simulink model "ADCS_MIL"  (R2024a)
settings: Solver=FixedStepAuto  StartTime=0.0  StopTime=6000  RelTol=1e-3
undefined symbols (not defined in the file or in its folder): agh, attitude, Cd, dgh, Eearth, epoch, Esun, Jsc, juliandate, k_Bdot, Kd1, Kd2, Kd3, km, Kp1, Kp2, Kp3, m, m_disturb, MTQ_Swithces, NoiseStd, s, satellite, signQuat, simulator, Surf_areas, Surf_dist, Surf_normals, Surf_reflectivity, WMM2020
libraries: sharedtransform x18, aerolibconvert2 x12, SepehrMILLib x11, simulink_extras x8, aerolibsatdyn x5, aerolibutil x5, sharedutil x3, vrlib x3, aerolibtransform2 x3, aerolibgravity2 x3, matrix_library x2
(part 1 of 3)
settings Model: Creator=dani  LastModifiedBy=dani

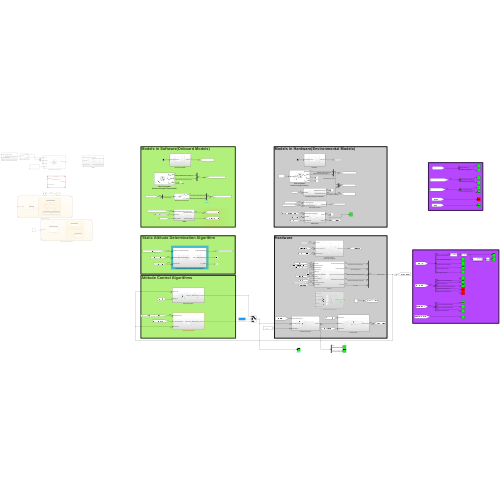
[thumbnail: Simulink's stored preview of the top-level diagram]
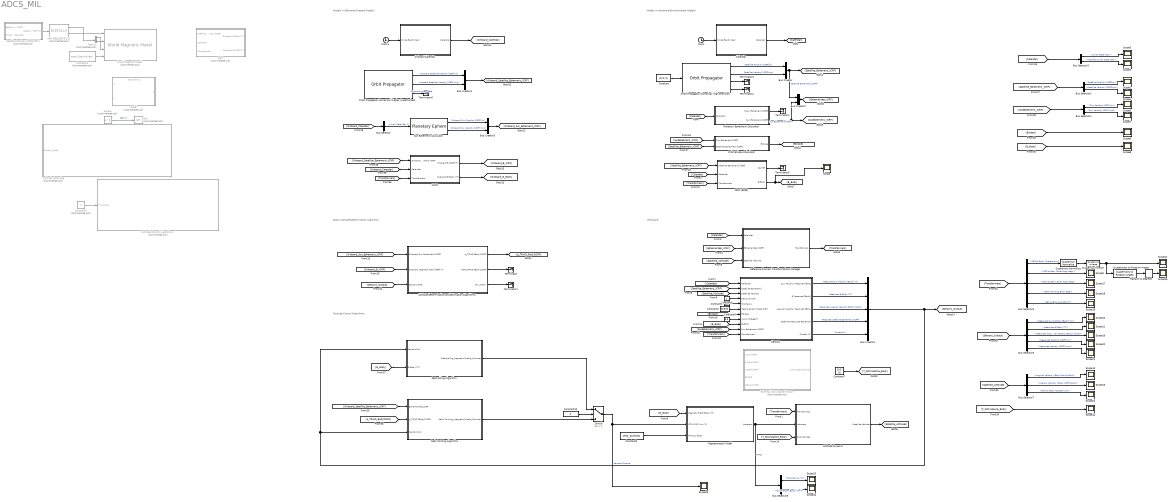
== system ADCS_MIL ==
  note: Hardware
  note: Models in Software(Onboard Models)
  note: Static Attitude Determination Algorithm
  note: Attitude Control Algorithms
  note: Models in Hardware(Environmental Models)
  Attitude Control Algorithms : Stateflow chart  Commented=on  TreatAsAtomicUnit=on
  Attitude Controlgg : Stateflow chart  Commented=on  TreatAsAtomicUnit=on
  Attitude Determination and Estimation Algorithms : Subsystem
  Attitude Dynamic : Subsystem
  Bus Creator{,2..4} (4 alike) : BusCreator  Inputs=2
  Bus Creator1 : BusCreator  Inputs=5
  Bus Selector : BusSelector  OutputSignals=Julian Date (day)
  Bus Selector2 : BusSelector  OutputSignals=Satellite Position [ICRF](m),Satellite Velocity [ICRF](m/s)
  Bus Selector3 : BusSelector  OutputSignals=Julian Date (day),Modified Julian Date (day)
  Bus Selector4 : BusSelector  OutputSignals=Sun Position [ICRF] (m),Sun Velocity [ICRF] (m/s)
  Bus Selector5 : BusSelector  OutputSignals=Measured Sun Position [Body] (m),Measured B [Body] (T),Measured Angular Velocity [Body] (rad/s),Measured Satellite Ephemeris [ICRF].Measured Position [ICRF] (m),Measured Satellite Ephemeris [ICRF].Measured Velocity [ICRF] (m/s)
  Bus Selector6 : BusSelector  OutputSignals=Quaternions.ICRF to Body Quaternions,Euler Angles (deg).ICRF to Body Euler Angs (deg),Euler Angles (deg).Orbit to Body Euler Angs (deg),Pinting Error (Deg).Nadir Pointing Error (deg),Orbital Elements.Semi-Major Axis [a] (m)
  Bus Selector7 : BusSelector  OutputSignals=Angular Velocity {Body-Orbit}(rad/s),Angular Velocity {Body-ICRF}(rad/s),Orbit to Body Quaternions
  Bus Selector8 : BusSelector  OutputSignals=Dipoles (Am^2),CoilsTorque [Body] (Nm)
  "Calendar " : Subsystem
  Clock : Clock
  Clock1 : Clock
  Constant : Constant  Value=[0; 0; 0]
  Constant1 : Constant  Value=20
  Constant10 : Constant  Value=0
  Constant2 : Constant  Value=eye(3)
  Constant3 : Constant  Commented=on  Value=epoch.DecimalYear
  Constant4 : Constant  Commented=on  Value=2
  Constant5 : Constant
  Constant6 : Constant  Value=3.3
  Constant7 : Constant  Value=[0 0 0]
  Constant9 : Constant  Value=MTQ_Swithces
  Demux : Demux  Commented=on  Outputs=2
  Detumbling Algorithm : Subsystem
  External Disturbance Torque : Subsystem  Commented=on
  IGRF : Subsystem  Commented=on
  IGRF [ECEF] : Subsystem
  ITRF Position to LLA : ECEF2LLA  Commented=on
  Magnetorquers Model : Subsystem
  Model : ModelReference  Commented=on  ModelNameDialog=Detumbling.slx  SimulationMode=Normal  ModelReferenceVersion=1.5
      settings: PortSchema="{\"entries\":[{\"content\":{\"sides\":[{\"content\":{\"connectorIds\":[\"In2\",\"In1\"]},\"type\":\"ConnectorPlacement.EquallySpacedRectSide\",\"uuid\":\"6955eca1-02f6-4ce4-b58e-cf6f86409957\"},{\"content\":{\"connectorIds\":[\"Out1\"],\"side\":\"RIGHT\"},\"type\":\"ConnectorPlacement.EquallySpacedRectSide\",\"uuid\":\"f24cf38f-2c71-460d-85e4-067bf27b1853\"},{\"content\":{\"side\":\"TOP\"},\"type\":\"ConnectorPlacement.EquallySpacedRectSide\",\"uuid\":\"bfc76406-ab18-49d9-8c0b-a4b5f97489f3\"}]},\"type\":\"ConnectorPlacement.EquallySpacedConnector\",\"uuid\":\"b367625e-d4b0-440c-86d9-252cf79ffd42\"}],\"packageUris\":[\"http://schema.mathworks.com/mf0/Connector/R2020b\"],\"version\":\"1.0\"}"
  Nadir Pointing Algorithm : Subsystem
  Onboard Calendar : Subsystem
  Orbit Eclipse Calculator : Subsystem
  Orbit Propagator Numerical (Kepler-Unperturbed) : OrbitPropagator  accelIn=on  startDate=juliandate(epoch.Year, epoch.Month, epoch.Day, epoch.Hour, epoch.Minute, epoch.Second)  orbitType=Circular inclined  semiMajorAxis=Semi_major_axis  inclination=Inclination  raan=RAAN  argLat=Argument_of_latitude  inertialPosition=[3649700.0 3308200.0 -4676600.0]  inertialVelocity=[-2750.8 6666.4 2573.4]  fixedPosition=[-4142689.0 -2676864.7 -4669861.6]  fixedVelocity=[1452.7 -6720.7 2568.1]  customR=3396200  customMu=4.305e13  customJ2=1.0826269e-03  customOmega=4.06125949e-3  outputTransform=on
  Orbit Propagator Numerical (high precision) : OrbitPropagator  propagator=Numerical (high precision)  accelIn=on  startDate=juliandate(epoch.Year, epoch.Month, epoch.Day, epoch.Hour, epoch.Minute, epoch.Second)  orbitType=Circular inclined  semiMajorAxis=Semi_major_axis  inclination=Inclination  raan=RAAN  argLat=Argument_of_latitude  inertialPosition=[3649700.0 3308200.0 -4676600.0]  inertialVelocity=[-2750.8 6666.4 2573.4]  fixedPosition=[-4142689.0 -2676864.7 -4669861.6]  fixedVelocity=[1452.7 -6720.7 2568.1]  customR=3396200  customMu=4.305e13  customJ2=1.0826269e-03  customOmega=4.06125949e-3  outputTransform=on
  Planetary Ephemeris Calculator : Subsystem
  Quaternion Inverse : aerolibutil/Quaternion Inverse
  Quaternion Normalize : sharedutil/Quaternion Normalize  aMode=aMode
  Quaternions to Rotation Angles : sharedtransform/Quaternions to Rotation Angles  rotationOrder=XYZ  aMode=aMode
  Radians to Degrees : simulink_extras/Transformations/Radians to Degrees
  Reference Frames Transformations Manager : Subsystem
  Satellite Position [ICRF2ITRF] : Subsystem  Commented=on
  Scope{,1..26} (27 alike) : Scope
  Sensors : Subsystem
  Sqrt : Sqrt  Commented=on
  Square : Math  Commented=on  Operator=square
  Sun Ephemeris Calculator : PlanetaryEphem  target=Sun
  Switch : Switch  Criteria=u2 > Threshold  Threshold=1  SaturateOnIntegerOverflow=off  InputSameDT=off
  Terminator{,1..6} (7 alike) : Terminator
  WMM : Subsystem
  World Magnetic Model : aerolibgravity2/World Magnetic Model  Commented=on  model=WMM2020 (2020-2025)  customFile='WMM2020.COF'  units=Metric (MKS)  time_in=on  month=January  day=1  year=2020  action=Error  h_out=off  dec_out=off  inc_out=off  ti_out=off
  wires:
  [Calendar] -> Sensors/1(Calendar)
  [Transformers] -> IGRF [ECEF]/3(Transformers)
  [Calendar] -> IGRF [ECEF]/2(Calendar)
  [Satellite_Attitude] -> Reference Frames Transformations Manager/3(Satellite Attitude)
  Sensors/2(B Measured [Body]) -> Bus Creator1/2  "Measured B [Body] (T)"
  Constant5/1 -> Sensors/4(Sensor Switch)
  [Ephemerides_ICRF] -> Reference Frames Transformations Manager/2(Ephemerides [ICRF])
  Attitude Dynamic/1(Satellite Attitude) -> [Satellite_Attitude]
  Constant9/1 -> Magnetorquers Model/3(MTQ Switches)
  [B_Body] -> Magnetorquers Model/1(Magnetic Field [Body] (T))
  Sensors/4(Satellite Measured Ephemeris) -> Bus Creator1/4  "Measured Satellite Ephemeris [ICRF]"
  Magnetorquers Model/1(Acutators) -> Bus Selector8/1, Attitude Dynamic/2(Actuators)  "MTQs"
  Sensors/3(Angular Velocity Measured [Body]) -> Bus Creator1/3  "Measured Angular Velocity [Body] (rad/s)"
  Sensors/1(Sun Position Measured [Body]) -> Bus Creator1/1  "Measured Sun Position [Body] (m)"
  "Calendar "/1(Calendar) -> [Calendar]
  Clock/1 -> "Calendar "/1(Since Epoch (sec))
  Reference Frames Transformations Manager/1(Transformers) -> [Transformers]
  Orbit Propagator Numerical (high precision)/2 -> Bus Creator/2  "Satellite Velocity [ICRF](m/s)"
  [Calendar] -> Planetary Ephemeris Calculator/1(Calendar)
  Orbit Propagator Numerical (high precision)/1 -> Bus Creator/1  "Satellite Position [ICRF](m)"
  Planetary Ephemeris Calculator/2(Sun Ephemeris [ICRF]) -> Bus Creator2/2, [SunEphemeris_ICRF]  "Sun Ephemeris [ICRF]"
  [Calendar] -> Reference Frames Transformations Manager/1(Calendar)
  Planetary Ephemeris Calculator/1(Moon Ephemeris [ICRF]) -> Terminator4/1
  [Transformers] -> Attitude Dynamic/1(Transformers)
  Constant7/1 -> [T_Distrubance_Body]
  Orbit Propagator Numerical (high precision)/4 -> Terminator2/1
  Constant1/1 -> Sensors/5(MM_Temp)
  [Satellite_Attitude] -> Sensors/3(Satellite Attitude)
  Constant2/1 -> Sensors/6(Measurement Model DCM)
  Constant/1 -> Orbit Propagator Numerical (high precision)/1
  [Satellite_Ephemeris_ICRF] -> Sensors/2(Satellite Ephemeris)
  Sensors/5(Current (A)) -> Bus Creator1/5  "Current (A)"
  [Eclipse] -> Sensors/7(Eclipse)
  [T_Distrubance_Body] -> Attitude Dynamic/3(Disturbances)
  Bus Creator1/1 -> [Sensors_Output], Detumbling Algorithm/1(Sensors Out), Nadir Pointing Algorithm/3(Sensors Out)  "Sensors Outputs"
  Orbit Propagator Numerical (high precision)/3 -> Terminator3/1
  Orbit Propagator Numerical (Kepler-Unperturbed)/1 -> Bus Creator4/1  "Onboard Satellite Position [ICRF] (m)"
  Attitude Determination and Estimation Algorithms/3(Cov_Matrix) -> Terminator1/1
  Attitude Determination and Estimation Algorithms/2(DCM_TRIAD [Body2ICRF]) -> Terminator/1
  Attitude Determination and Estimation Algorithms/1(q_TRIAD [Body2ICRF]) -> [q_TRIAD_Body2ICRF]
  IGRF [ECEF]/2(B_Body) -> Scope/1, [B_Body]
  IGRF [ECEF]/1(B_ITRF) -> Terminator5/1
  [B_Body] -> Sensors/9(B_Body)
  Constant4/1 -> Attitude Control Algorithms/1(Sys_Mode)
  [SunEphemeris_ICRF] -> Orbit Eclipse Calculator/1(Sun Ephemeris [ICRF])
  [Satellite_Ephemeris_ICRF] -> Orbit Eclipse Calculator/2(Satellite Ephemeris [ICRF])
  Orbit Eclipse Calculator/1(Eclipse) -> [Eclipse]
  Bus Creator/1 -> Bus Creator2/1, [Satellite_Ephemeris_ICRF]  "Satellite Ephemeris [ICRF]"
  [Satellite_Ephemeris_ICRF] -> IGRF [ECEF]/1(Satellite Ephemeris [ICRF])
  Bus Creator2/1 -> [Ephemerides_ICRF]
  Constant6/1 -> Sensors/8(Input Voltage(V))
  Sun Ephemeris Calculator/1 -> Bus Creator3/1  "Onboard Sun Position [ICRF] (m)"
  Sun Ephemeris Calculator/2 -> Bus Creator3/2  "Onboard Sun Velocity [ICRF] (m/s)"
  Bus Creator3/1 -> [Onboard_Sun_Ephemeris_ICRF]
  Orbit Propagator Numerical (Kepler-Unperturbed)/2 -> Bus Creator4/2  "Onboard Satellite Velocity [ICRF] (m/s)"
  Bus Creator4/1 -> [Onboard_Satellite_Ephemeris_ICRF]
  [Onboard_Calendar] -> Bus Selector/1
  Bus Selector/1 -> Sun Ephemeris Calculator/1  "<Julian Date (day)>"
  Clock1/1 -> Onboard Calendar/1(Since Epoch (sec))
  Onboard Calendar/1(Calendar) -> [Onboard_Calendar]
  Orbit Propagator Numerical (Kepler-Unperturbed)/3 -> Terminator6/1  "Onboard Julian Date"
  [SunEphemeris_ICRF] -> Sensors/10(Sun Ephemeris [ICRF])
  [Transformers] -> Sensors/11(Transformers)
  [Onboard_Sun_Ephemeris_ICRF] -> Attitude Determination and Estimation Algorithms/1(Onboard Sun Ephemeris [ICRF])
  [Calendar] -> Bus Selector3/1
  [Satellite_Ephemeris_ICRF] -> Bus Selector2/1
  [SunEphemeris_ICRF] -> Bus Selector4/1
  [Eclipse] -> Scope6/1
  Bus Selector3/1 -> Scope3/1  "<Julian Date (day)>"
  Bus Selector3/2 -> Scope1/1  "<Modified Julian Date (day)>"
  Bus Selector2/1 -> Scope2/1  "<Satellite Position [ICRF](m)>"
  Bus Selector2/2 -> Scope4/1  "<Satellite Velocity [ICRF](m/s)>"
  Bus Selector4/2 -> Scope7/1  "<Sun Velocity [ICRF] (m/s)>"
  Bus Selector4/1 -> Scope5/1  "<Sun Position [ICRF] (m)>"
  [B_Body] -> Scope8/1
  Bus Selector6/1 -> Quaternion Normalize/1  "<ICRF to Body Quaternions>"
  Bus Selector6/2 -> Scope9/1  "<ICRF to Body Euler Angs (deg)>"
  [Sensors_Output] -> Bus Selector5/1
  Bus Selector5/2 -> Scope12/1  "<Measured B [Body] (T)>"
  [Satellite_Attitude] -> Bus Selector7/1
  [T_Distrubance_Body] -> Scope14/1
  Bus Selector5/1 -> Scope10/1  "<Measured Sun Position [Body] (m)>"
  [Transformers] -> Bus Selector6/1
  Bus Selector7/1 -> Scope13/1  "<Angular Velocity {Body-Orbit}(rad/s)>"
  Bus Selector7/2 -> Scope15/1  "<Angular Velocity {Body-ICRF}(rad/s)>"
  Bus Selector6/3 -> Scope17/1  "<Orbit to Body Euler Angs (deg)>"
  Bus Selector6/4 -> Scope18/1  "<Nadir Pointing Error (deg)>"
  Bus Selector6/5 -> Scope19/1  "<Semi-Major Axis [a] (m)>"
  Bus Selector5/3 -> Scope16/1  "<Measured Angular Velocity [Body] (rad/s)>"
  Bus Selector5/5 -> Scope21/1  "<Measured Velocity [ICRF] (m/s)>"
  Bus Selector5/4 -> Scope20/1  "<Measured Position [ICRF] (m)>"
  Bus Selector7/3 -> Scope22/1  "<Orbit to Body Quaternions>"
  Square/1 -> Sqrt/1  "||B||^2"
  Bus Selector8/1 -> Scope23/1  "<Dipoles (Am^2)>"
  Bus Selector8/2 -> Scope24/1  "<CoilsTorque [Body] (Nm)>"
  Constant10/1 -> Switch/2
  Switch/1 -> Scope25/1, Magnetorquers Model/2(MTQ CMD (A.m^2))
  Detumbling Algorithm/1(Detumbling_Magnetic Dipole_Command) -> Switch/1
  [Onboard_Satellite_Ephemeris_ICRF] -> Nadir Pointing Algorithm/1(Ephemerides_ICRF)
  [B_Body] -> Detumbling Algorithm/2(B [Body] (T))
  [q_TRIAD_Body2ICRF] -> Nadir Pointing Algorithm/2(q_TRIAD [Body2ICRF])
  Quaternion Normalize/1 -> Quaternion Inverse/1
  Quaternion Inverse/1 -> Quaternions to Rotation Angles/1, Scope11/1
  Quaternions to Rotation Angles/1 -> Radians to Degrees/1
  Radians to Degrees/1 -> Scope26/1
  [Transformers] -> WMM/3(Transformers)
  [Onboard_Calendar] -> WMM/2(Calendar)
  [Onboard_Satellite_Ephemeris_ICRF] -> WMM/1(Onboard Satellite Ephemeris [ICRF])
  ITRF Position to LLA/1 -> Demux/1
  Satellite Position [ICRF2ITRF]/1(Satellite Position [ITRF] (m)) -> ITRF Position to LLA/1
  Demux/2 -> World Magnetic Model/3
  Demux/1 -> World Magnetic Model/2
  ITRF Position to LLA/2 -> World Magnetic Model/1
  Constant3/1 -> World Magnetic Model/4
  WMM/1(Onboard B [ICRF] (T)) -> [Onboard_B_ICRF]
  [Sensors_Output] -> Attitude Determination and Estimation Algorithms/3(Sensors Data)
  [Onboard_B_ICRF] -> Attitude Determination and Estimation Algorithms/2(Onboard Magnetic Field [ICRF] (T))
  WMM/2(Onboard B [Body] (T)) -> [Onboard_B_Body]
  Nadir Pointing Algorithm/1(Nadir Pointing_Magnetic Dipole_Command) -> Switch/3

== system ADCS_MIL/Attitude Control Algorithms/Off ==
  Sys_Mode : Inport
  Action Port : ActionPort
      settings: CopyFcn=Stateflow.SLINSF.SimulinkMan.removeBlockPreDeleteFcn  PreDeleteFcn=Stateflow.SLINSF.SimulinkMan.unsafePredeleteFcn

== system ADCS_MIL/Attitude Control Algorithms/On.Detumbling ==
  Sys_Mode : Inport
  Action Port : ActionPort
      settings: CopyFcn=Stateflow.SLINSF.SimulinkMan.removeBlockPreDeleteFcn  PreDeleteFcn=Stateflow.SLINSF.SimulinkMan.unsafePredeleteFcn
  Model : ModelReference  ModelNameDialog=Detumbling.slx  SimulationMode=Normal  ModelReferenceVersion=1.1
  Terminator : Terminator
  wires:
  Sys_Mode/1 -> Terminator/1

== system ADCS_MIL/Attitude Control Algorithms/On.Nadir_Pointing ==
  Sys_Mode : Inport
  q_TRIAD : Inport  Port=2
  Action Port : ActionPort
      settings: CopyFcn=Stateflow.SLINSF.SimulinkMan.removeBlockPreDeleteFcn  PreDeleteFcn=Stateflow.SLINSF.SimulinkMan.unsafePredeleteFcn

== system ADCS_MIL/Attitude Controlgg/Off ==
  SensorsOut : Inport  OutDataTypeStr=Bus: StatesOutBus
  " " : ActionPort
      settings: CopyFcn=Stateflow.SLINSF.SimulinkMan.removeBlockPreDeleteFcn  PreDeleteFcn=Stateflow.SLINSF.SimulinkMan.unsafePredeleteFcn
  Terminator : Terminator
  TorqueCmds : Constant  Value=[0 0 0]
  Unit quat : Constant  Value=[1 0 0 0]
  PointingCmd : Outport  VectorParamsAs1DForOutWhenUnconnected=off
  cmd_q_b2tgt : Outport  Port=2  VectorParamsAs1DForOutWhenUnconnected=off
  wires:
  SensorsOut/1 -> Terminator/1
  TorqueCmds/1 -> PointingCmd/1  "torque_cmds"
  Unit quat/1 -> cmd_q_b2tgt/1  "torque_cmds"

== system ADCS_MIL/Attitude Controlgg/On.Detumbling ==
  SensorsOut : Inport  OutDataTypeStr=Bus: StatesOutBus
  Environment : Inport  Port=2  OutDataTypeStr=Bus: EnvBus
  " " : ActionPort
      settings: CopyFcn=Stateflow.SLINSF.SimulinkMan.removeBlockPreDeleteFcn  PreDeleteFcn=Stateflow.SLINSF.SimulinkMan.unsafePredeleteFcn
  Attitude Profile (Sun Tracking) : aerolibsatdyn/Attitude Profile (Nadir Pointing)  outputError=on  outputFinalAttitude=off  portFrame=ICRF  pointingMode=Custom  celestialTarget=Sun  tunablePointing=off  primaryAlignmentSrc=Dialog  primaryAlignment=[0 0 -1]  secondaryAlignmentSrc=Dialog  secondaryAlignment=[1 0 0]  constraintFrame=ICRF  primaryConstraintSrc=Port  primaryConstraint=[1 0 0]  secondaryConstraintSrc=Dialog  secondaryConstraint=[0 0 1]
  Bus Selector : BusSelector  OutputSignals=x_sun_eci
  Bus Selector1 : BusSelector  OutputSignals=X_eci,q_eci2b
  Model : ModelReference  ModelNameDialog=Detumbling.slx  SimulationMode=Normal  ModelReferenceVersion=1.1
  Quaternion Conjugate : aerolibutil/Quaternion Conjugate
  Quaternions to Rotation Angles1 : sharedtransform/Quaternions to Rotation Angles  rotationOrder=XYZ  aMode=aMode
  PointingCmd : Outport  VectorParamsAs1DForOutWhenUnconnected=off
  cmd_q_b2tgt : Outport  Port=2  VectorParamsAs1DForOutWhenUnconnected=off
  wires:
  Attitude Profile (Sun Tracking)/1 -> Quaternions to Rotation Angles1/1, cmd_q_b2tgt/1
  SensorsOut/1 -> Bus Selector1/1
  Environment/1 -> Bus Selector/1
  Quaternions to Rotation Angles1/1 -> PointingCmd/1
  Bus Selector/1 -> Attitude Profile (Sun Tracking)/3  "<x_sun_eci>"
  Quaternion Conjugate/1 -> Attitude Profile (Sun Tracking)/2
  Bus Selector1/2 -> Quaternion Conjugate/1  "<q_eci2b>"
  Bus Selector1/1 -> Attitude Profile (Sun Tracking)/1  "<X_eci>"

== system ADCS_MIL/Attitude Controlgg/On.Nadir_Pointing ==
  SensorsOut : Inport  OutDataTypeStr=Bus: StatesOutBus
  " " : ActionPort
      settings: CopyFcn=Stateflow.SLINSF.SimulinkMan.removeBlockPreDeleteFcn  PreDeleteFcn=Stateflow.SLINSF.SimulinkMan.unsafePredeleteFcn
  Attitude Profile (Nadir Pointing) : aerolibsatdyn/Attitude Profile (Nadir Pointing)  outputError=on  outputFinalAttitude=off  portFrame=ICRF  pointingMode=Point at nadir  celestialTarget=Sun  tunablePointing=off  primaryAlignmentSrc=Dialog  primaryAlignment=[0 0 1]  secondaryAlignmentSrc=Dialog  secondaryAlignment=[1 0 0]  constraintFrame=LVLH  primaryConstraintSrc=Dialog  primaryConstraint=[1 0 0]  secondaryConstraintSrc=Dialog  secondaryConstraint=[0 1 0]
  Bus Selector : BusSelector  OutputSignals=X_eci,V_eci,q_eci2b
  Nadir Pointing : Subsystem
  Quaternion Conjugate : aerolibutil/Quaternion Conjugate
  Quaternions to Rotation Angles : sharedtransform/Quaternions to Rotation Angles  rotationOrder=XYZ  aMode=aMode
  PointingCmd : Outport  VectorParamsAs1DForOutWhenUnconnected=off
  cmd_q_b2tgt : Outport  Port=2  VectorParamsAs1DForOutWhenUnconnected=off
  Out1 : Outport  Port=3
  wires:
  Quaternions to Rotation Angles/1 -> PointingCmd/1
  Bus Selector/3 -> Quaternion Conjugate/1  "<q_eci2b>"
  Bus Selector/2 -> Attitude Profile (Nadir Pointing)/2  "<V_eci>"
  SensorsOut/1 -> Bus Selector/1
  Bus Selector/1 -> Attitude Profile (Nadir Pointing)/1  "<X_eci>"
  Quaternion Conjugate/1 -> Attitude Profile (Nadir Pointing)/3
  Attitude Profile (Nadir Pointing)/1 -> cmd_q_b2tgt/1, Quaternions to Rotation Angles/1
  Nadir Pointing/1(m_Command) -> Out1/1

== system ADCS_MIL/Attitude Controlgg/On.Sun_Pointing ==
  SensorsOut : Inport  OutDataTypeStr=Bus: StatesOutBus
  Environment : Inport  Port=2  OutDataTypeStr=Bus: EnvBus
  " " : ActionPort
      settings: CopyFcn=Stateflow.SLINSF.SimulinkMan.removeBlockPreDeleteFcn  PreDeleteFcn=Stateflow.SLINSF.SimulinkMan.unsafePredeleteFcn
  Attitude Profile (Sun Tracking) : aerolibsatdyn/Attitude Profile (Nadir Pointing)  outputError=on  outputFinalAttitude=off  portFrame=ICRF  pointingMode=Custom  celestialTarget=Sun  tunablePointing=off  primaryAlignmentSrc=Dialog  primaryAlignment=[0 0 -1]  secondaryAlignmentSrc=Dialog  secondaryAlignment=[1 0 0]  constraintFrame=ICRF  primaryConstraintSrc=Port  primaryConstraint=[1 0 0]  secondaryConstraintSrc=Dialog  secondaryConstraint=[0 0 1]
  Bus Selector : BusSelector  OutputSignals=x_sun_eci
  Bus Selector1 : BusSelector  OutputSignals=X_eci,q_eci2b
  Quaternion Conjugate : aerolibutil/Quaternion Conjugate
  Quaternions to Rotation Angles1 : sharedtransform/Quaternions to Rotation Angles  rotationOrder=XYZ  aMode=aMode
  PointingCmd : Outport  VectorParamsAs1DForOutWhenUnconnected=off
  cmd_q_b2tgt : Outport  Port=2  VectorParamsAs1DForOutWhenUnconnected=off
  wires:
  Attitude Profile (Sun Tracking)/1 -> Quaternions to Rotation Angles1/1, cmd_q_b2tgt/1
  SensorsOut/1 -> Bus Selector1/1
  Environment/1 -> Bus Selector/1
  Quaternions to Rotation Angles1/1 -> PointingCmd/1
  Bus Selector/1 -> Attitude Profile (Sun Tracking)/3  "<x_sun_eci>"
  Quaternion Conjugate/1 -> Attitude Profile (Sun Tracking)/2
  Bus Selector1/2 -> Quaternion Conjugate/1  "<q_eci2b>"
  Bus Selector1/1 -> Attitude Profile (Sun Tracking)/1  "<X_eci>"

== system ADCS_MIL/Attitude Determination and Estimation Algorithms ==
  Onboard Sun Ephemeris [ICRF] : Inport
  Onboard Magnetic Field [ICRF] (T) : Inport  Port=2
  Sensors Data : Inport  Port=3
  Bus Selector : BusSelector  OutputSignals=Measured Sun Position [Body] (m),Measured B [Body] (T)
  Bus Selector1 : BusSelector  OutputSignals=Onboard Sun Position [ICRF] (m)
  Constant : Constant  Value=NoiseStd
  Constant1 : Constant  Value=signQuat
  MATLAB Function1 : MATLAB Function  TreatAsAtomicUnit=on
  Quaternion Normalize : sharedutil/Quaternion Normalize  aMode=aMode
  q_TRIAD [Body2ICRF] : Outport
  DCM_TRIAD [Body2ICRF] : Outport  Port=2
  Cov_Matrix : Outport  Port=3
  wires:
  MATLAB Function1/1(quat_TRIAD) -> Quaternion Normalize/1
  MATLAB Function1/2(CovarianceMatrix) -> Cov_Matrix/1
  MATLAB Function1/3(RotationMatrix) -> DCM_TRIAD [Body2ICRF]/1
  Sensors Data/1 -> Bus Selector/1
  Bus Selector/1 -> MATLAB Function1/3(SunPos_Body)  "<Measured Sun Position [Body] (m)>"
  Bus Selector/2 -> MATLAB Function1/4(MagField_Body)  "<Measured B [Body] (T)>"
  Constant/1 -> MATLAB Function1/5(NoiseStd)
  Constant1/1 -> MATLAB Function1/6(signQuat)
  Onboard Sun Ephemeris [ICRF]/1 -> Bus Selector1/1
  Bus Selector1/1 -> MATLAB Function1/1(SunPos_ECI)  "<Onboard Sun Position [ICRF] (m)>"
  Onboard Magnetic Field [ICRF] (T)/1 -> MATLAB Function1/2(MagField_ECI)
  Quaternion Normalize/1 -> q_TRIAD [Body2ICRF]/1

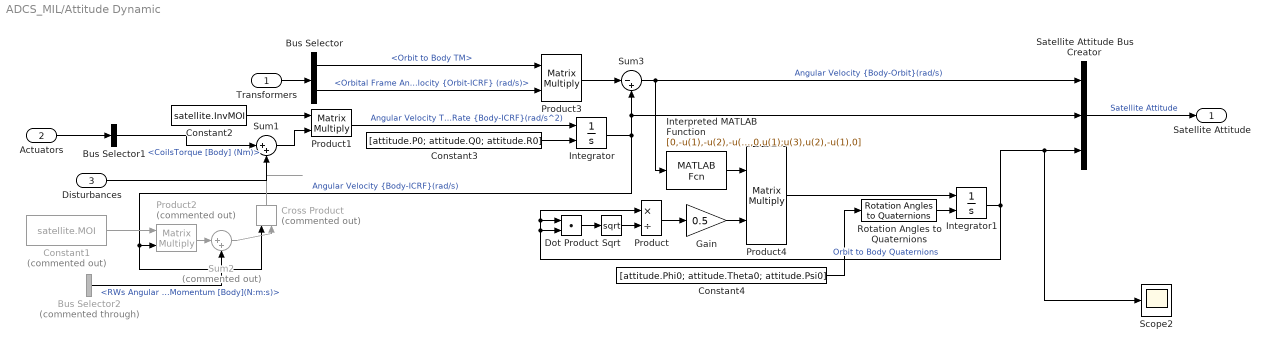
== system ADCS_MIL/Attitude Dynamic ==
  Transformers : Inport
  Actuators : Inport  Port=2
  Disturbances : Inport  Port=3
  Bus Selector : BusSelector  OutputSignals=Transfer Matrices.Orbit to Body TM,Orbital Elements.Orbital Frame Angular Velocity {Orbit-ICRF} (rad/s)
  Bus Selector1 : BusSelector  OutputSignals=CoilsTorque [Body] (Nm)
  Bus Selector2 : BusSelector  Commented=through  OutputSignals=Momenta [Body].RWs Angular Momentum [Body](N:m:s)
  Constant1 : Constant  Commented=on  Value=satellite.MOI
  Constant2 : Constant  Value=satellite.InvMOI
  Constant3 : Constant  Value=[attitude.P0; attitude.Q0; attitude.R0]
  Constant4 : Constant  Value=[attitude.Phi0; attitude.Theta0; attitude.Psi0]
  Cross Product : vrlib/Utilities/Cross Product  Commented=on
  Dot Product : DotProduct  OutDataTypeStr=Inherit: Inherit via internal rule
  Gain : Gain  Gain=0.5
  Integrator : Integrator  InitialConditionSource=external  ContinuousStateAttributes={'P','Q','R'}
  Integrator1 : Integrator  InitialConditionSource=external  ContinuousStateAttributes={'q0','q1','q2','q3'}
  Interpreted MATLAB Function : MATLABFcn  MATLABFcn=[0,-u(1),-u(2),-u(3);u(1),0,u(3),-u(2);u(2),-u(3),0,u(1);u(3),u(2),-u(1),0]  OutputDimensions=[4,4]  OutputSignalType=real  Output1D=off
  Product : Product  Inputs=*/
  Product1 : Product  Multiplication=Matrix(*)
  Product2 : Product  Commented=on  Multiplication=Matrix(*)
  Product3 : Product  Multiplication=Matrix(*)
  Product4 : Product  Multiplication=Matrix(*)
  Rotation Angles to Quaternions : sharedtransform/Rotation Angles to Quaternions  rotationOrder=XYZ  aMode=aMode
  Satellite Attitude Bus Creator : BusCreator  Inputs=3
  Scope2 : Scope
  Sqrt : Sqrt  OutputSignalType=real
  Sum1 : Sum  Inputs=|++
  Sum2 : Sum  Commented=on  Inputs=|++
  Sum3 : Sum  Inputs=|-+
  Satellite Attitude : Outport
  wires:
  Integrator/1 -> Product2/2, Cross Product/1, Satellite Attitude Bus Creator/2, Sum3/2  "Angular Velocity {Body-ICRF}(rad/s)"
  Bus Selector/2 -> Product3/2  "<Orbital Frame Angular Velocity {Orbit-ICRF} (rad/s)>"
  Constant2/1 -> Product1/1
  Interpreted MATLAB Function/1 -> Product4/1
  Bus Selector1/1 -> Sum1/1  "<CoilsTorque [Body] (Nm)>"
  Constant1/1 -> Product2/1
  Dot Product/1 -> Sqrt/1
  Sqrt/1 -> Product/2
  Sum2/1 -> Cross Product/2
  Satellite Attitude Bus Creator/1 -> Satellite Attitude/1  "Satellite Attitude"
  Product3/1 -> Sum3/1
  Sum1/1 -> Product1/2
  Constant4/1 -> Rotation Angles to Quaternions/1
  Bus Selector2/1 -> Sum2/2  "<RWs Angular Momentum [Body](N:m:s)>"
  Cross Product/1 -> ?
  Transformers/1 -> Bus Selector/1
  Product1/1 -> Integrator/1  "Angular Velocity Time Rate {Body-ICRF}(rad/s^2)"
  Gain/1 -> Product4/2
  Constant3/1 -> Integrator/2
  Product4/1 -> Integrator1/1
  Bus Selector/1 -> Product3/1  "<Orbit to Body TM>"
  Integrator1/1 -> Dot Product/2, Product/1, Dot Product/1, Scope2/1, Satellite Attitude Bus Creator/3  "Orbit to Body Quaternions"
  Product2/1 -> Sum2/1
  Sum3/1 -> Satellite Attitude Bus Creator/1, Interpreted MATLAB Function/1  "Angular Velocity {Body-Orbit}(rad/s)"
  Actuators/1 -> Bus Selector1/1
  Rotation Angles to Quaternions/1 -> Integrator1/2
  Product/1 -> Gain/1
  Disturbances/1 -> Sum1/2

== system ADCS_MIL/Calendar  ==
  Since Epoch (sec) : Inport  OutDataTypeStr=double  Unit=s  PortDimensions=1
  Calendar Bus Creator : BusCreator  Inputs=4
  Constant6 : Constant  Value=epoch.DecimalYear
  JD : Subsystem
  MJD : Subsystem
  Calendar : Outport
  wires:
  Since Epoch (sec)/1 -> MJD/1(Since Epoch (sec)), JD/1(Since Epoch (sec)), Calendar Bus Creator/4  "Since Epoch (sec)"
  Constant6/1 -> Calendar Bus Creator/3  "Decimal Year (year)"
  JD/1(Julian Date (day)) -> Calendar Bus Creator/1  "Julian Date (day)"
  Calendar Bus Creator/1 -> Calendar/1  "Calendar_out"
  MJD/1(Modified Julian Date (day)) -> Calendar Bus Creator/2  "Modified Julian Date (day)"

== system ADCS_MIL/Detumbling Algorithm ==
  Sensors Out : Inport
  B [Body] (T) : Inport  Port=2
  Abs : Abs  SaturateOnIntegerOverflow=off
  Bus Selector1 : BusSelector  OutputSignals=Measured Angular Velocity [Body] (rad/s)
  Constant11 : Constant  Value=k_Bdot
  Cross Product : matrix_library/Cross Product
  Cross Product1 : matrix_library/Cross Product
  Demux : Demux  Outputs=3
  Divide : Product  Inputs=*/
  Divide1 : Product  Inputs=*/
  MATLAB Function : MATLAB Function  TreatAsAtomicUnit=on
  Mux : Mux  Inputs=3
  Saturation : Saturate  UpperLimit=5  LowerLimit=-5
  Saturation1 : Saturate  UpperLimit=5  LowerLimit=-5
  Saturation2 : Saturate  UpperLimit=5  LowerLimit=-5
  Scope : Scope
  Scope1 : Scope
  Scope2 : Scope
  Detumbling_Magnetic Dipole_Command : Outport
  wires:
  MATLAB Function/1(length) -> Divide1/2, Scope1/1, Divide/2  "||B||"
  Divide1/1 -> Demux/1  "k/||B||*omega*b"
  Cross Product1/1 -> Divide1/1  "k*omega*b"
  Cross Product/1 -> Cross Product1/2  "omega*b"
  Divide/1 -> Cross Product/2  "b"
  Sensors Out/1 -> Bus Selector1/1
  Abs/1 -> Scope/1
  B [Body] (T)/1 -> Abs/1, MATLAB Function/1(vector), Divide/1
  Bus Selector1/1 -> Cross Product/1  "<Measured Angular Velocity [Body] (rad/s)>"
  Demux/2 -> Saturation/1
  Demux/1 -> Saturation1/1
  Demux/3 -> Saturation2/1
  Saturation/1 -> Mux/2
  Saturation2/1 -> Mux/3
  Saturation1/1 -> Mux/1
  Mux/1 -> Scope2/1, Detumbling_Magnetic Dipole_Command/1
  Constant11/1 -> Cross Product1/1

== system ADCS_MIL/External Disturbance Torque ==
  R_Sun[ICRF] : Inport
  R_Earth[ICRF] : Inport  Port=2
  V_Earth[ICRF] : Inport  Port=3
  B[ICRF] : Inport  Port=4
  q[Body2ICRF] : Inport  Port=5
  Absolute values : MATLAB Function  TreatAsAtomicUnit=on
  Drag : Subsystem
  Gravitional : Subsystem
  Magnetic : Subsystem
  Radiation Pressure : Subsystem
  Scope : Scope
  Scope3 : Scope
  Sum1 : Sum  Inputs=++++
  Terminator : Terminator
  Terminator1 : Terminator
  T_disturbance_Total : Outport
  wires:
  Magnetic/3(Magnetic torque) -> Absolute values/1(s1), Sum1/1
  q[Body2ICRF]/1 -> Magnetic/3(Abn), Radiation Pressure/3(Abn), Drag/3(Abn), Gravitional/3(Abn)
  Drag/1(Drag torque) -> Absolute values/3(s3), Sum1/3
  Sum1/1 -> Scope/1, T_disturbance_Total/1
  Magnetic/1(Bn) -> Terminator/1
  Magnetic/2(Bb) -> Terminator1/1
  V_Earth[ICRF]/1 -> Gravitional/2(Vsc_earth), Drag/2(Vsc_earth)
  Absolute values/1(st) -> Scope3/1
  Gravitional/1(Grav torque) -> Absolute values/4(s4), Sum1/4
  Radiation Pressure/1(RP torque) -> Absolute values/2(s2), Sum1/2
  B[ICRF]/1 -> Magnetic/2(Earth RA)
  R_Earth[ICRF]/1 -> Magnetic/1(Rsc_earth), Radiation Pressure/2(Rsc_earth), Gravitional/1(Rsc_earth), Drag/1(Rsc_earth)
  R_Sun[ICRF]/1 -> Radiation Pressure/1(Rsc_sun)

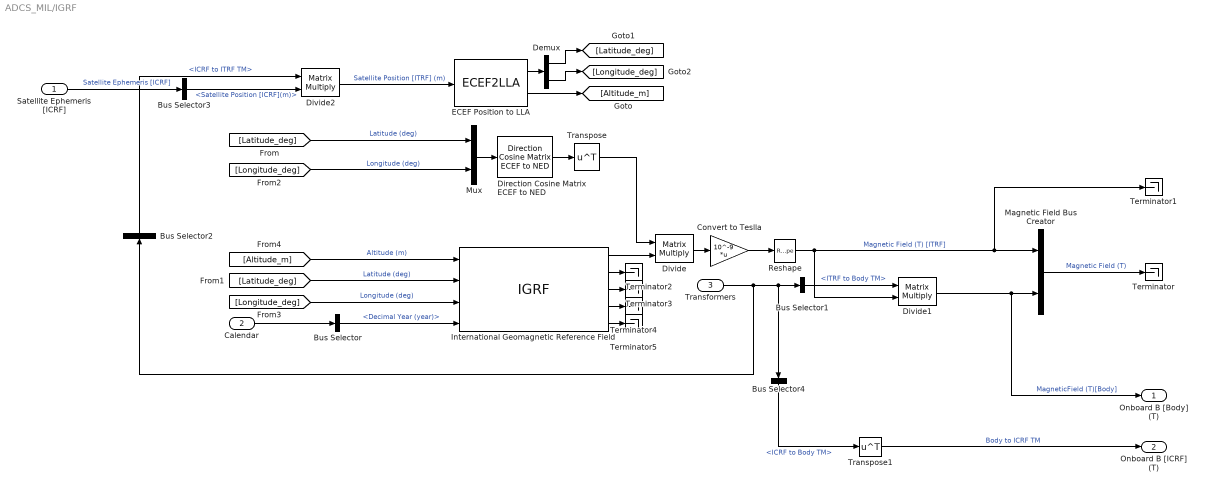
== system ADCS_MIL/IGRF ==
  Satellite Ephemeris [ICRF] : Inport
  Calendar : Inport  Port=2
  Transformers : Inport  Port=3
  Bus Selector : BusSelector  OutputSignals=Decimal Year (year)
  Bus Selector1 : BusSelector  OutputSignals=Transfer Matrices.ITRF to Body TM
  Bus Selector2 : BusSelector  OutputSignals=Transfer Matrices.ICRF to ITRF TM
  Bus Selector3 : BusSelector  OutputSignals=Satellite Position [ICRF](m)
  Bus Selector4 : BusSelector  OutputSignals=Transfer Matrices.ICRF to Body TM
  Convert to Teslla : Gain  Gain=10^-9  Multiplication=Matrix(K*u)
  Demux : Demux  Outputs=2
  Direction Cosine Matrix ECEF to NED : aerolibtransform2/Direction Cosine Matrix ECEF to NED
  Divide : Product  Inputs=**  Multiplication=Matrix(*)
  Divide1 : Product  Inputs=**  Multiplication=Matrix(*)
  Divide2 : Product  Inputs=**  Multiplication=Matrix(*)
  ECEF Position to LLA : ECEF2LLA
  International Geomagnetic Reference Field : IGRF  month=January  day=1  year=2020  sv_out=off
      settings: AttributesFormatString=%<generation>
  Magnetic Field Bus Creator : BusCreator  Inputs=2
  Mux : Mux  Inputs=2
  Reshape : Reshape  OutputDimensionality=Customize  OutputDimensions=[3,1]
  Terminator{,1..5} (6 alike) : Terminator
  Transpose : Math  Operator=transpose
  Transpose1 : Math  Operator=transpose
  Onboard B [Body] (T) : Outport
  Onboard B [ICRF] (T) : Outport  Port=2
  wires:
  [Latitude_deg] -> International Geomagnetic Reference Field/2  "Latitude (deg)"
  Transpose/1 -> Divide/1
  Demux/1 -> [Latitude_deg]
  [Altitude_m] -> International Geomagnetic Reference Field/1  "Altitude (m)"
  Reshape/1 -> Terminator1/1, Magnetic Field Bus Creator/1, Divide1/2  "Magnetic Field (T) [ITRF]"
  Direction Cosine Matrix ECEF to NED/1 -> Transpose/1
  Magnetic Field Bus Creator/1 -> Terminator/1  "Magnetic Field (T)"
  Mux/1 -> Direction Cosine Matrix ECEF to NED/1
  Transformers/1 -> Bus Selector1/1, Bus Selector4/1, Bus Selector2/1
  [Latitude_deg] -> Mux/1  "Latitude (deg)"
  [Longitude_deg] -> Mux/2  "Longitude (deg)"
  ECEF Position to LLA/2 -> [Altitude_m]
  Demux/2 -> [Longitude_deg]
  Divide/1 -> Convert to Teslla/1
  Convert to Teslla/1 -> Reshape/1
  Calendar/1 -> Bus Selector/1
  ECEF Position to LLA/1 -> Demux/1
  Divide2/1 -> ECEF Position to LLA/1  "Satellite Position [ITRF] (m)"
  [Longitude_deg] -> International Geomagnetic Reference Field/3  "Longitude (deg)"
  Bus Selector/1 -> International Geomagnetic Reference Field/4  "<Decimal Year (year)>"
  Divide1/1 -> Onboard B [Body] (T)/1, Magnetic Field Bus Creator/2  "MagneticField (T)[Body]"
  International Geomagnetic Reference Field/1 -> Divide/2
  Bus Selector1/1 -> Divide1/1  "<ITRF to Body TM>"
  Satellite Ephemeris [ICRF]/1 -> Bus Selector3/1  "Satellite Ephemeris [ICRF]"
  Bus Selector2/1 -> Divide2/1  "<ICRF to ITRF TM>"
  Bus Selector3/1 -> Divide2/2  "<Satellite Position [ICRF](m)>"
  Bus Selector4/1 -> Transpose1/1  "<ICRF to Body TM>"
  Transpose1/1 -> Onboard B [ICRF] (T)/1  "Body to ICRF TM"
  International Geomagnetic Reference Field/5 -> Terminator5/1
  International Geomagnetic Reference Field/4 -> Terminator4/1
  International Geomagnetic Reference Field/3 -> Terminator3/1
  International Geomagnetic Reference Field/2 -> Terminator2/1

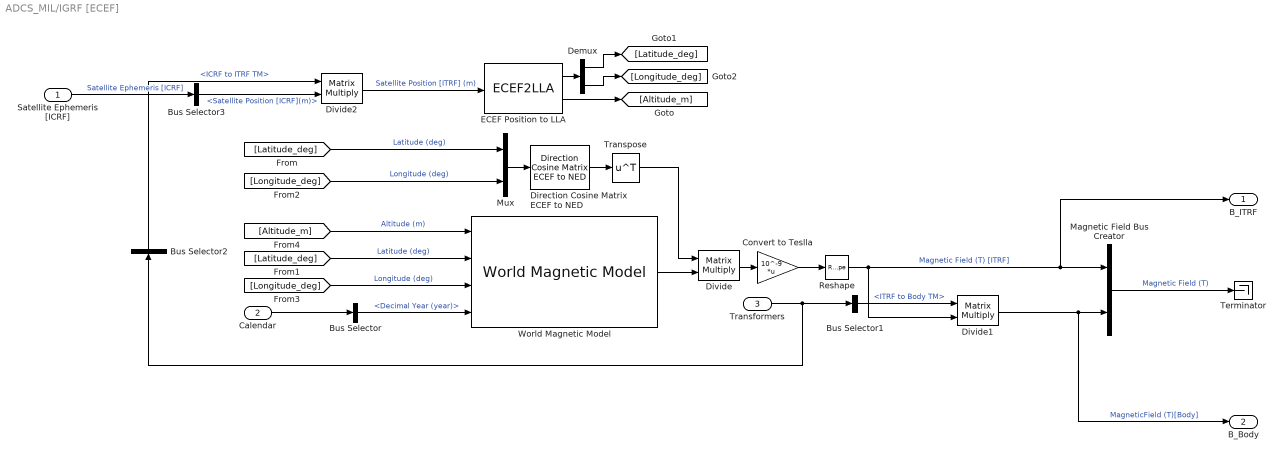
== system ADCS_MIL/IGRF [ECEF] ==
  Satellite Ephemeris [ICRF] : Inport
  Calendar : Inport  Port=2
  Transformers : Inport  Port=3
  Bus Selector : BusSelector  OutputSignals=Decimal Year (year)
  Bus Selector1 : BusSelector  OutputSignals=Transfer Matrices.ITRF to Body TM
  Bus Selector2 : BusSelector  OutputSignals=Transfer Matrices.ICRF to ITRF TM
  Bus Selector3 : BusSelector  OutputSignals=Satellite Position [ICRF](m)
  Convert to Teslla : Gain  Gain=10^-9  Multiplication=Matrix(K*u)
  Demux : Demux  Outputs=2
  Direction Cosine Matrix ECEF to NED : aerolibtransform2/Direction Cosine Matrix ECEF to NED
  Divide : Product  Inputs=**  Multiplication=Matrix(*)
  Divide1 : Product  Inputs=**  Multiplication=Matrix(*)
  Divide2 : Product  Inputs=**  Multiplication=Matrix(*)
  ECEF Position to LLA : ECEF2LLA
  Magnetic Field Bus Creator : BusCreator  Inputs=2
  Mux : Mux  Inputs=2
  Reshape : Reshape  OutputDimensionality=Customize  OutputDimensions=[3,1]
  Terminator : Terminator
  Transpose : Math  Operator=transpose
  World Magnetic Model : aerolibgravity2/World Magnetic Model  model=WMM2020 (2020-2025)  customFile='WMM2020.COF'  units=Metric (MKS)  time_in=on  month=January  day=1  year=2020  action=Error  h_out=off  dec_out=off  inc_out=off  ti_out=off
  B_ITRF : Outport
  B_Body : Outport  Port=2
  wires:
  [Latitude_deg] -> World Magnetic Model/2  "Latitude (deg)"
  Transpose/1 -> Divide/1
  Demux/1 -> [Latitude_deg]
  [Altitude_m] -> World Magnetic Model/1  "Altitude (m)"
  Reshape/1 -> B_ITRF/1, Magnetic Field Bus Creator/1, Divide1/2  "Magnetic Field (T) [ITRF]"
  Direction Cosine Matrix ECEF to NED/1 -> Transpose/1
  Magnetic Field Bus Creator/1 -> Terminator/1  "Magnetic Field (T)"
  Mux/1 -> Direction Cosine Matrix ECEF to NED/1
  Transformers/1 -> Bus Selector1/1, Bus Selector2/1
  [Latitude_deg] -> Mux/1  "Latitude (deg)"
  [Longitude_deg] -> Mux/2  "Longitude (deg)"
  ECEF Position to LLA/2 -> [Altitude_m]
  Demux/2 -> [Longitude_deg]
  Divide/1 -> Convert to Teslla/1
  Convert to Teslla/1 -> Reshape/1
  Calendar/1 -> Bus Selector/1
  ECEF Position to LLA/1 -> Demux/1
  Divide2/1 -> ECEF Position to LLA/1  "Satellite Position [ITRF] (m)"
  [Longitude_deg] -> World Magnetic Model/3  "Longitude (deg)"
  Bus Selector/1 -> World Magnetic Model/4  "<Decimal Year (year)>"
  Divide1/1 -> B_Body/1, Magnetic Field Bus Creator/2  "MagneticField (T)[Body]"
  World Magnetic Model/1 -> Divide/2
  Bus Selector1/1 -> Divide1/1  "<ITRF to Body TM>"
  Satellite Ephemeris [ICRF]/1 -> Bus Selector3/1  "Satellite Ephemeris [ICRF]"
  Bus Selector2/1 -> Divide2/1  "<ICRF to ITRF TM>"
  Bus Selector3/1 -> Divide2/2  "<Satellite Position [ICRF](m)>"

== system ADCS_MIL/Magnetorquers Model ==
  Magnetic Field [Body] (T) : Inport
  MTQ CMD (A.m^2) : Inport  Port=2  PortDimensions=[3,1]
  MTQ Switches : Inport  Port=3  PortDimensions=[3,1]
  Abs : Abs  SaturateOnIntegerOverflow=off
  Abs1 : Abs  SaturateOnIntegerOverflow=off
  Constant : Constant
  Constant1 : Constant
  Cross Product : vrlib/Utilities/Cross Product
  Dot Product : DotProduct  OutDataTypeStr=Inherit: Inherit via internal rule
  Gain : Gain  Gain=0.5
  Gain1 : Gain  Gain=-1
  Gain2 : Gain  Gain=0.5
  Magnetorquers Bus Creator : BusCreator  Inputs=3
  Nominal Dipole : Constant  Value=satellite.MTQ.DPMoment
  Nominal Dipole1 : Constant  Value=satellite.MTQ.DPMoment
  Power : Constant  Value=satellite.MTQ.Power
  Product : Product  Inputs=3
  Product1 : Product  Inputs=*/
  Product2 : Product
  Product3 : Product
  Sign : Signum
  Sign1 : Signum
  Sign2 : Signum
  Sum : Sum  Inputs=|+-
  Sum1 : Sum  Inputs=|++
  Sum2 : Sum  Inputs=++|
  Sum3 : Sum  Inputs=|++
  Acutators : Outport
  wires:
  Product3/1 -> Product1/1, Sign1/1, Product2/1, Abs/1
  Product2/1 -> Sum3/1
  Product1/1 -> Abs1/1
  Gain/1 -> Product/2
  Abs1/1 -> Dot Product/1
  Product/1 -> Sum3/2
  Sum1/1 -> Gain/1
  Nominal Dipole/1 -> Product/3, Sum/2
  Sign/1 -> Sum1/1
  Dot Product/1 -> Magnetorquers Bus Creator/3  "Power (W)"
  Magnetic Field [Body] (T)/1 -> Cross Product/2
  Abs/1 -> Sum/1
  MTQ Switches/1 -> Product3/2
  Gain2/1 -> Product2/2
  Power/1 -> Dot Product/2
  Sum3/1 -> Magnetorquers Bus Creator/1, Cross Product/1  "Dipoles (Am^2)"
  Nominal Dipole1/1 -> Product1/2
  Sum2/1 -> Gain2/1
  Sign2/1 -> Sum2/2
  Constant1/1 -> Sum2/1
  Sum/1 -> Sign/1, Gain1/1
  MTQ CMD (A.m^2)/1 -> Product3/1
  Magnetorquers Bus Creator/1 -> Acutators/1  "Actuators"
  Constant/1 -> Sum1/2
  Cross Product/1 -> Magnetorquers Bus Creator/2  "CoilsTorque [Body] (Nm)"
  Sign1/1 -> Product/1
  Gain1/1 -> Sign2/1

== system ADCS_MIL/Nadir Pointing Algorithm ==
  Ephemerides_ICRF : Inport
  q_TRIAD [Body2ICRF] : Inport  Port=2
  Sensors Out : Inport  Port=3
  -Kd1 : Gain  Gain=-1 * Kd1
  -Kd2 : Gain  Gain=-1 * Kd2
  -Kd3 : Gain  Gain=-1 * Kd3
  -Kp1 : Gain  Gain=-1 * Kp1
  -Kp2 : Gain  Gain=-1 * Kp2
  -Kp3 : Gain  Gain=-1 * Kp3
  Bus Selector1 : BusSelector  OutputSignals=Measured Angular Velocity [Body] (rad/s)
  Demux : Demux
  Demux1 : Demux  Outputs=3
  Mux : Mux  Inputs=3
  PD Controller : Subsystem  Commented=on
  Quaternion Normalize1 : sharedutil/Quaternion Normalize  aMode=aMode
  Saturation : Saturate  UpperLimit=5  LowerLimit=-5
  Saturation1 : Saturate  UpperLimit=5  LowerLimit=-5
  Saturation2 : Saturate  UpperLimit=5  LowerLimit=-5
  Scope2 : Scope
  Scope3 : Scope
  Sum1 : Sum  Inputs=|++
  Sum2 : Sum  Inputs=|++
  Sum3 : Sum  Inputs=|++
  Terminator : Terminator
  q_Desired Propagator : Subsystem
  q_error Calculator : Subsystem
  Nadir Pointing_Magnetic Dipole_Command : Outport
  wires:
  Ephemerides_ICRF/1 -> q_Desired Propagator/1(Satellite Ephemeris)
  Bus Selector1/1 -> Demux1/1  "<Measured Angular Velocity [Body] (rad/s)>"
  q_Desired Propagator/1(q_Desired) -> q_error Calculator/1(q_Desired)
  q_TRIAD [Body2ICRF]/1 -> q_error Calculator/2(q_Real), q_Desired Propagator/2(q [Body2ICRF])  "Body to ICRF Quaternion"
  Sensors Out/1 -> Bus Selector1/1
  q_error Calculator/1(q_Error) -> Quaternion Normalize1/1, Scope3/1
  Demux/2 -> -Kp1/1
  Demux/1 -> Terminator/1
  Demux/3 -> -Kp2/1
  Demux/4 -> -Kp3/1
  Quaternion Normalize1/1 -> Demux/1
  -Kp1/1 -> Sum1/2
  -Kp2/1 -> Sum2/2
  -Kp3/1 -> Sum3/2
  Demux1/1 -> -Kd1/1
  Demux1/2 -> -Kd2/1
  Demux1/3 -> -Kd3/1
  -Kd1/1 -> Sum1/1
  -Kd2/1 -> Sum2/1
  -Kd3/1 -> Sum3/1
  Sum1/1 -> Saturation/1  "m1"
  Sum2/1 -> Saturation1/1  "m2"
  Sum3/1 -> Saturation2/1  "m3"
  Saturation1/1 -> Mux/2
  Saturation/1 -> Mux/1
  Saturation2/1 -> Mux/3
  Mux/1 -> Scope2/1, Nadir Pointing_Magnetic Dipole_Command/1

== system ADCS_MIL/Onboard Calendar ==
  Since Epoch (sec) : Inport  OutDataTypeStr=double  Unit=s  PortDimensions=1
  Calendar Bus Creator : BusCreator  Inputs=4
  Constant6 : Constant  Value=epoch.DecimalYear
  JD : Subsystem
  MJD : Subsystem
  Calendar : Outport
  wires:
  Since Epoch (sec)/1 -> MJD/1(Since Epoch (sec)), JD/1(Since Epoch (sec)), Calendar Bus Creator/4  "Since Epoch (sec)"
  Constant6/1 -> Calendar Bus Creator/3  "Decimal Year (year)"
  JD/1(Julian Date (day)) -> Calendar Bus Creator/1  "Julian Date (day)"
  Calendar Bus Creator/1 -> Calendar/1  "Calendar_out"
  MJD/1(Modified Julian Date (day)) -> Calendar Bus Creator/2  "Modified Julian Date (day)"

== system ADCS_MIL/Orbit Eclipse Calculator ==
  Sun Ephemeris [ICRF] : Inport
  Satellite Ephemeris [ICRF] : Inport  Port=2
  Atan2 : Trigonometry  Operator=atan2
  Bus Selector : BusSelector  OutputSignals=Satellite Position [ICRF](m)
  Bus Selector1 : BusSelector  OutputSignals=Sun Position [ICRF] (m)
  MATLAB Function1 : MATLAB Function  Commented=on  TreatAsAtomicUnit=on
  Eclipse : Outport
  wires:
  Sun Ephemeris [ICRF]/1 -> Bus Selector1/1
  Satellite Ephemeris [ICRF]/1 -> Bus Selector/1
  Atan2/1 -> Eclipse/1  "Alpha"
  Bus Selector/1 -> Atan2/2  "<Satellite Position [ICRF](m)>"
  MATLAB Function1/1(Eclipse) -> ?
  Bus Selector1/1 -> Atan2/1  "<Sun Position [ICRF] (m)>"

== system ADCS_MIL/Planetary Ephemeris Calculator ==
  Calendar : Inport
  Bus Selector : BusSelector  OutputSignals=Julian Date (day)
  Length Conversion : aerolibconvert2/Length Conversion  IU=km  OU=m
  Length Conversion1 : aerolibconvert2/Length Conversion  IU=km  OU=m
  Moon Ephemeris Bus Creator : BusCreator  Inputs=2
  Moon Ephemeris Calculator : PlanetaryEphem
  Sun Ephemeris Bus Creator : BusCreator  Inputs=2
  Sun Ephemeris Calculator : PlanetaryEphem  target=Sun
  Velocity Conversion : aerolibconvert2/Velocity Conversion  IU=km/s  OU=m/s
  Velocity Conversion1 : aerolibconvert2/Velocity Conversion  IU=km/s  OU=m/s
  Moon Ephemeris [ICRF] : Outport
  Sun Ephemeris [ICRF] : Outport  Port=2
  wires:
  Moon Ephemeris Bus Creator/1 -> Moon Ephemeris [ICRF]/1  "Moon Ephemeris [ICRF]"
  Velocity Conversion/1 -> Moon Ephemeris Bus Creator/2  "Moon Velocity [ICRF] (m/s)"
  Bus Selector/1 -> Moon Ephemeris Calculator/1, Sun Ephemeris Calculator/1  "<Julian Date (day)>"
  Moon Ephemeris Calculator/2 -> Velocity Conversion/1
  Calendar/1 -> Bus Selector/1
  Sun Ephemeris Calculator/1 -> Length Conversion1/1
  Sun Ephemeris Calculator/2 -> Velocity Conversion1/1
  Velocity Conversion1/1 -> Sun Ephemeris Bus Creator/2  "Sun Velocity [ICRF] (m/s)"
  Length Conversion/1 -> Moon Ephemeris Bus Creator/1  "Moon Position [ICRF] (m)"
  Sun Ephemeris Bus Creator/1 -> Sun Ephemeris [ICRF]/1  "Sun Ephemeris [ICRF]"
  Length Conversion1/1 -> Sun Ephemeris Bus Creator/1  "Sun Position [ICRF] (m)"
  Moon Ephemeris Calculator/1 -> Length Conversion/1
